simulink model "NNPID_Control"  (R2023a)
settings: Solver=VariableStepAuto  StartTime=0.0  StopTime=5  RelTol=1e-3
settings Model: Creator=24731  LastModifiedBy=24731
settings DebuggingCC: AlgebraicLoopMsg=none

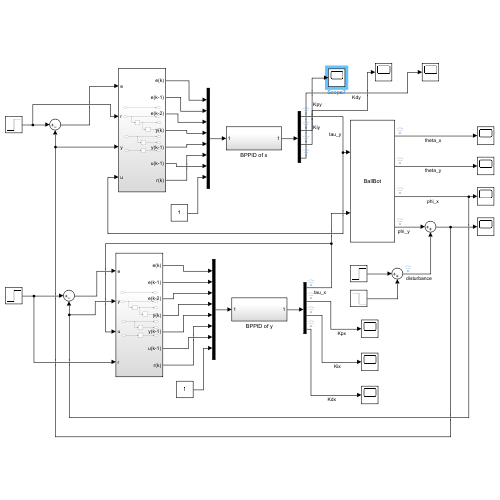
[thumbnail: Simulink's stored preview of the top-level diagram]
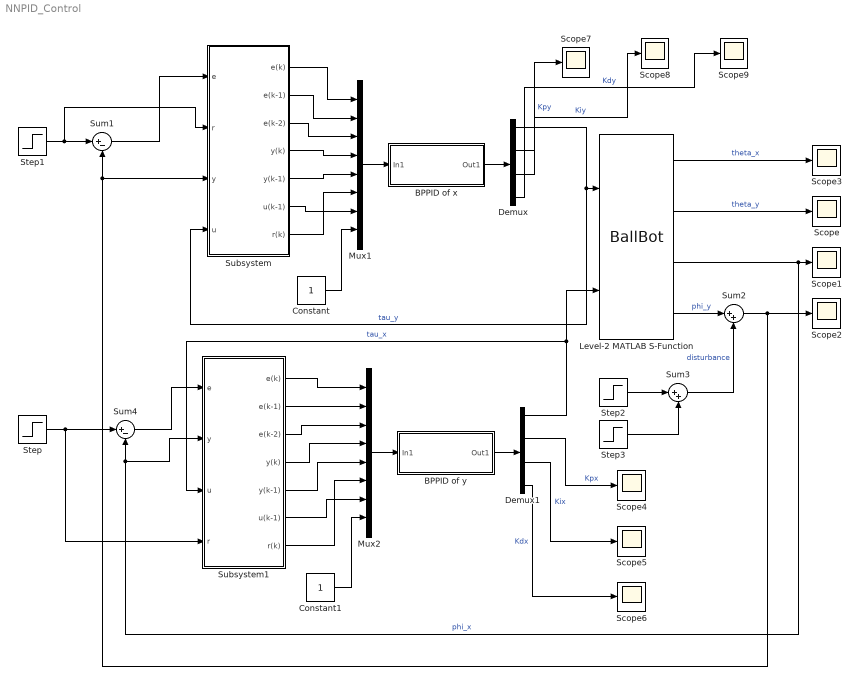
== system NNPID_Control ==
  "BPPID of x " : Subsystem
  BPPID of y : Subsystem
  Constant : Constant
  Constant1 : Constant
  Demux : Demux
  Demux1 : Demux
  Level-2 MATLAB S-Function : M-S-Function  FunctionName=BallBot  Parameters=0;0;-0.1;0.1;0;0;0;0
  Mux1 : Mux  Inputs=8
  Mux2 : Mux  Inputs=8
  Scope{,1..9} (10 alike) : Scope
  Step : Step  Time=0  After=0  SampleTime=0.01
  Step1 : Step  Time=0  After=0  SampleTime=0.01
  Step2 : Step  Time=3  After=0.05  SampleTime=0
  Step3 : Step  Time=3.1  After=-0.05  SampleTime=0
  Subsystem : Subsystem
  Subsystem1 : Subsystem
  Sum1 : Sum  Inputs=|+-
  Sum2 : Sum  Inputs=|++
  Sum3 : Sum  Inputs=|++
  Sum4 : Sum  Inputs=|+-
  wires:
  Level-2 MATLAB S-Function/2 -> Scope/1  "theta_y"
  Level-2 MATLAB S-Function/4 -> Sum2/1  "phi_y"
  Step1/1 -> Sum1/1, Subsystem/2(r)
  Sum2/1 -> Scope2/1, Subsystem/3(y), Sum1/2
  Level-2 MATLAB S-Function/3 -> Scope1/1, Subsystem1/2(y), Sum4/2  "phi_x"
  Sum3/1 -> Sum2/2  "disturbance"
  Level-2 MATLAB S-Function/1 -> Scope3/1  "theta_x"
  "BPPID of x "/1(Out1) -> Demux/1
  Step3/1 -> Sum3/2
  Sum1/1 -> Subsystem/1(e)
  Step2/1 -> Sum3/1
  Mux1/1 -> "BPPID of x "/1(In1)
  Subsystem/1(e(k)) -> Mux1/1
  Subsystem/2(e(k-1)) -> Mux1/2
  Subsystem/3(e(k-2)) -> Mux1/3
  Subsystem/4(y(k)) -> Mux1/4
  Subsystem/5(y(k-1)) -> Mux1/5
  Subsystem/7(r(k)) -> Mux1/6
  Subsystem/6(u(k-1)) -> Mux1/7
  Constant/1 -> Mux1/8
  Subsystem1/2(e(k-1)) -> Mux2/2
  Subsystem1/3(e(k-2)) -> Mux2/3
  Sum4/1 -> Subsystem1/1(e)
  Subsystem1/1(e(k)) -> Mux2/1
  Step/1 -> Sum4/1, Subsystem1/4(r)
  Subsystem1/7(r(k)) -> Mux2/6
  Subsystem1/5(y(k-1)) -> Mux2/5
  Subsystem1/6(u(k-1)) -> Mux2/7
  Constant1/1 -> Mux2/8
  Demux1/1 -> Subsystem1/3(u), Level-2 MATLAB S-Function/2  "tau_x"
  BPPID of y/1(Out1) -> Demux1/1
  Mux2/1 -> BPPID of y/1(In1)
  Subsystem1/4(y(k)) -> Mux2/4
  Demux1/2 -> Scope4/1  "Kpx"
  Demux1/3 -> Scope5/1  "Kix"
  Demux1/4 -> Scope6/1  "Kdx"
  Demux/1 -> Level-2 MATLAB S-Function/1, Subsystem/4(u)  "tau_y"
  Demux/2 -> Scope7/1  "Kpy"
  Demux/3 -> Scope8/1  "Kiy"
  Demux/4 -> Scope9/1  "Kdy"

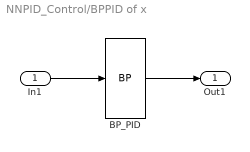
== system NNPID_Control/BPPID of x  ==
  In1 : Inport
  BP_PID : S-Function  FunctionName=BP  SFunctionDeploymentMode=off  EnableBusSupport=off
  Out1 : Outport
  wires:
  In1/1 -> BP_PID/1
  BP_PID/1 -> Out1/1

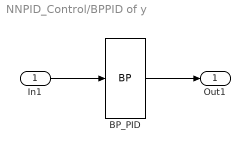
== system NNPID_Control/BPPID of y ==
  In1 : Inport
  BP_PID : S-Function  FunctionName=BP  SFunctionDeploymentMode=off  EnableBusSupport=off
  Out1 : Outport
  wires:
  In1/1 -> BP_PID/1
  BP_PID/1 -> Out1/1

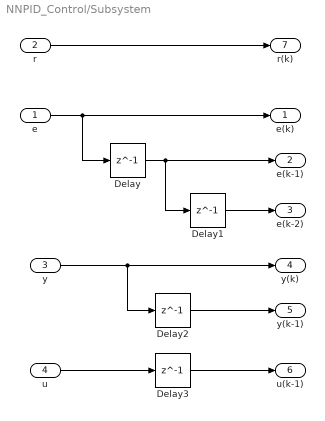
== system NNPID_Control/Subsystem ==
  e : Inport
  r : Inport  Port=2
  y : Inport  Port=3
  u : Inport  Port=4
  Delay{,1..3} (4 alike) : Delay  DelayLength=1  InitialCondition=0
  e(k) : Outport
  e(k-1) : Outport  Port=2
  e(k-2) : Outport  Port=3
  y(k) : Outport  Port=4
  y(k-1) : Outport  Port=5
  u(k-1) : Outport  Port=6
  r(k) : Outport  Port=7
  wires:
  e/1 -> Delay/1, e(k)/1
  Delay3/1 -> u(k-1)/1
  u/1 -> Delay3/1
  y/1 -> Delay2/1, y(k)/1
  Delay2/1 -> y(k-1)/1
  Delay1/1 -> e(k-2)/1
  Delay/1 -> Delay1/1, e(k-1)/1
  r/1 -> r(k)/1

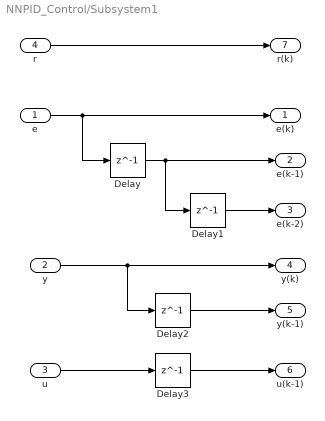
== system NNPID_Control/Subsystem1 ==
  e : Inport
  y : Inport  Port=2
  u : Inport  Port=3
  r : Inport  Port=4
  Delay{,1..3} (4 alike) : Delay  DelayLength=1  InitialCondition=0
  e(k) : Outport
  e(k-1) : Outport  Port=2
  e(k-2) : Outport  Port=3
  y(k) : Outport  Port=4
  y(k-1) : Outport  Port=5
  u(k-1) : Outport  Port=6
  r(k) : Outport  Port=7
  wires:
  e/1 -> Delay/1, e(k)/1
  Delay3/1 -> u(k-1)/1
  u/1 -> Delay3/1
  y/1 -> Delay2/1, y(k)/1
  Delay2/1 -> y(k-1)/1
  Delay1/1 -> e(k-2)/1
  Delay/1 -> Delay1/1, e(k-1)/1
  r/1 -> r(k)/1
